simulink model "TV_Controller"  (R2019b)
settings: Solver=VariableStepAuto  StartTime=0.0  StopTime=10.0  RelTol=1e-3
values from neighbouring files (symbols this model uses):
  Kd_wheelSlip = 0    [runTorqueVectoringScript.m]
  Kd_yawController = 0    [runTorqueVectoringScript.m]
  Ki_wheelSlip = 0.1    [runTorqueVectoringScript.m]
  Ki_yawController = 0.1    [runTorqueVectoringScript.m]
  Kp_wheelSlip = 10    [runTorqueVectoringScript.m]
  Kp_yawController = 10    [runTorqueVectoringScript.m]
  lambda = 0.5    [runTorqueVectoringScript.m]
  Rd = 0.2    [runTorqueVectoringScript.m]
  ref_slip = 0.11    [runTorqueVectoringScript.m]
  tr = 1.1    [runTorqueVectoringScript.m]
libraries: simulink x5
settings Model: Creator=mha483  LastModifiedBy=mha483

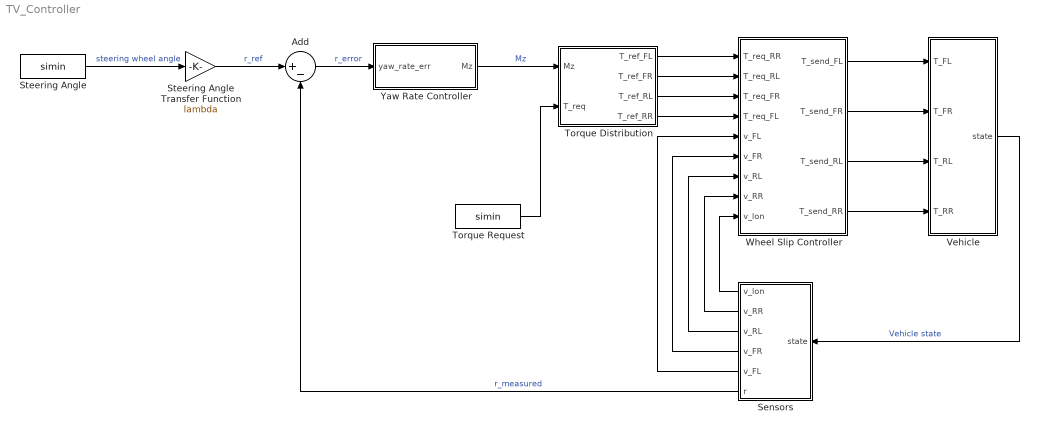
== system TV_Controller ==
  Add : Sum  Inputs=|+-
  Sensors : MATLAB Function  TreatAsAtomicUnit=on
  Steering Angle : FromWorkspace  VariableName=simin  SampleTime=0  Interpolate=off
  Steering Angle Transfer Function : Gain  Gain=lambda
  Torque Distribution : Subsystem
  Torque Request : FromWorkspace  VariableName=simin  SampleTime=0
  Vehicle : MATLAB Function  TreatAsAtomicUnit=on
  Wheel Slip Controller : Subsystem
  "Yaw Rate Controller " : Subsystem
  wires:
  "Yaw Rate Controller "/1(Mz) -> Torque Distribution/1(Mz)  "Mz"
  Torque Distribution/1(T_ref_FL) -> Wheel Slip Controller/1(T_req_RR)
  Torque Distribution/2(T_ref_FR) -> Wheel Slip Controller/2(T_req_RL)
  Torque Distribution/3(T_ref_RL) -> Wheel Slip Controller/3(T_req_FR)
  Torque Distribution/4(T_ref_RR) -> Wheel Slip Controller/4(T_req_FL)
  Add/1 -> "Yaw Rate Controller "/1(yaw_rate_err)  "r_error"
  Wheel Slip Controller/1(T_send_FL) -> Vehicle/1(T_FL)
  Wheel Slip Controller/2(T_send_FR) -> Vehicle/2(T_FR)
  Wheel Slip Controller/3(T_send_RL) -> Vehicle/3(T_RL)
  Wheel Slip Controller/4(T_send_RR) -> Vehicle/4(T_RR)
  Sensors/1(v_lon) -> Wheel Slip Controller/9(v_lon)
  Sensors/2(v_RR) -> Wheel Slip Controller/8(v_RR)
  Sensors/3(v_RL) -> Wheel Slip Controller/7(v_RL)
  Sensors/4(v_FR) -> Wheel Slip Controller/6(v_FR)
  Sensors/5(v_FL) -> Wheel Slip Controller/5(v_FL)
  Sensors/6(r) -> Add/2  "r_measured"
  Vehicle/1(state) -> Sensors/1(state)  "Vehicle state"
  Torque Request/1 -> Torque Distribution/2(T_req)
  Steering Angle Transfer Function/1 -> Add/1  "r_ref"
  Steering Angle/1 -> Steering Angle Transfer Function/1  "steering wheel angle"

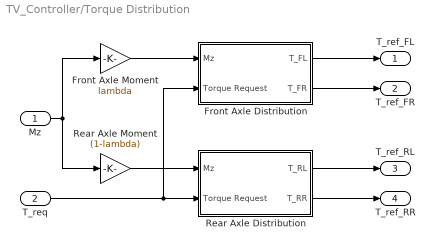
== system TV_Controller/Torque Distribution ==
  Mz : Inport
  T_req : Inport  Port=2
  Front Axle Moment : Gain  Gain=lambda
  Front Axle Distribution : Subsystem
  Rear Axle Moment : Gain  Gain=(1-lambda)
  Rear Axle Distribution : Subsystem
  T_ref_FL : Outport
  T_ref_FR : Outport  Port=2
  T_ref_RL : Outport  Port=3
  T_ref_RR : Outport  Port=4
  wires:
  Mz/1 -> Rear Axle Moment/1, Front Axle Moment/1
  Front Axle Moment/1 -> Front Axle Distribution/1(Mz)
  T_req/1 -> Rear Axle Distribution/2(Torque Request), Front Axle Distribution/2(Torque Request)
  Front Axle Distribution/2(T_FR) -> T_ref_FR/1
  Front Axle Distribution/1(T_FL) -> T_ref_FL/1
  Rear Axle Moment/1 -> Rear Axle Distribution/1(Mz)
  Rear Axle Distribution/1(T_RL) -> T_ref_RL/1
  Rear Axle Distribution/2(T_RR) -> T_ref_RR/1

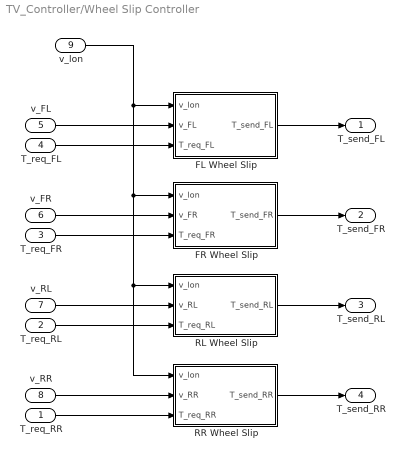
== system TV_Controller/Wheel Slip Controller ==
  T_req_RR : Inport
  T_req_RL : Inport  Port=2
  T_req_FR : Inport  Port=3
  T_req_FL : Inport  Port=4
  v_FL : Inport  Port=5
  v_FR : Inport  Port=6
  v_RL : Inport  Port=7
  v_RR : Inport  Port=8
  v_lon : Inport  Port=9
  FL Wheel Slip : Subsystem
  FR Wheel Slip : Subsystem
  RL Wheel Slip : Subsystem
  RR Wheel Slip : Subsystem
  T_send_FL : Outport
  T_send_FR : Outport  Port=2
  T_send_RL : Outport  Port=3
  T_send_RR : Outport  Port=4
  wires:
  v_lon/1 -> RR Wheel Slip/1(v_lon), RL Wheel Slip/1(v_lon), FR Wheel Slip/1(v_lon), FL Wheel Slip/1(v_lon)
  v_FL/1 -> FL Wheel Slip/2(v_FL)
  T_req_FL/1 -> FL Wheel Slip/3(T_req_FL)
  v_FR/1 -> FR Wheel Slip/2(v_FR)
  T_req_FR/1 -> FR Wheel Slip/3(T_req_FR)
  v_RL/1 -> RL Wheel Slip/2(v_RL)
  T_req_RL/1 -> RL Wheel Slip/3(T_req_RL)
  v_RR/1 -> RR Wheel Slip/2(v_RR)
  T_req_RR/1 -> RR Wheel Slip/3(T_req_RR)
  FL Wheel Slip/1(T_send_FL) -> T_send_FL/1
  FR Wheel Slip/1(T_send_FR) -> T_send_FR/1
  RL Wheel Slip/1(T_send_RL) -> T_send_RL/1
  RR Wheel Slip/1(T_send_RR) -> T_send_RR/1

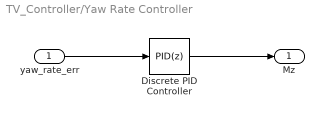
== system TV_Controller/Yaw Rate Controller  ==
  yaw_rate_err : Inport
  Discrete PID Controller : simulink/Continuous/PID Controller  Controller=PID  Form=Parallel  TimeDomain=Discrete-time  SampleTime=-1  IntegratorMethod=Forward Euler  FilterMethod=Forward Euler  ControllerParametersSource=internal  P=Kp_yawController  I=Ki_yawController  D=Kd_yawController  UseFilter=on  N=100  TunerSelectOption=Transfer Function Based (PID Tuner App)  InitialConditionSource=internal  InitialConditionForIntegrator=0  InitialConditionForFilter=0  DifferentiatorICPrevScaledInput=0  ExternalReset=none  TrackingMode=off  Kt=1  LimitOutput=off  UpperSaturationLimit=inf  LowerSaturationLimit=-inf  LinearizeAsGain=off  AntiWindupMode=none  Kb=1  POutMin=[]  POutMax=[]  IOutMin=[]  IOutMax=[]  DOutMin=[]  DOutMax=[]  NOutMin=[]  NOutMax=[]  SumOutMin=[]  SumOutMax=[]  SaturationOutMin=[]  SaturationOutMax=[]  PParamMin=[]  PParamMax=[]  IParamMin=[]  IParamMax=[]  DParamMin=[]  DParamMax=[]  NParamMin=[]  NParamMax=[]  KbParamMin=[]  KbParamMax=[]  KtParamMin=[]  KtParamMax=[]  KbOutMin=[]  KbOutMax=[]  KtOutMin=[]  KtOutMax=[]  IntegratorOutMin=[]  IntegratorOutMax=[]  FilterOutMin=[]  FilterOutMax=[]  SumI1OutMin=[]  SumI1OutMax=[]  SumI2OutMin=[]  SumI2OutMax=[]  SumI3OutMin=[]  SumI3OutMax=[]  SumI4OutMin=[]  SumI4OutMax=[]  SumDOutMin=[]  SumDOutMax=[]  DifferentiatorOutMin=[]  DifferentiatorOutMax=[]  FilterDiffOutCoefMin=[]  FilterDiffOutCoefMax=[]  ReciprocalOutMin=[]  ReciprocalOutMax=[]  SumDenOutMin=[]  SumDenOutMax=[]  SumNumOutMin=[]  SumNumOutMax=[]  DivideOutMin=[]  DivideOutMax=[]  IntegratorContinuousStateAttributes=''  IntegratorStateMustResolveToSignalObject=off  IntegratorRTWStateStorageClass=Auto  FilterContinuousStateAttributes=''  FilterStateMustResolveToSignalObject=off  FilterRTWStateStorageClass=Auto  ParallelPVariant=InternalParameters  IdealPVariant=Disabled  IVariant=InternalParameters  DVariant=InternalParameters  IntegratorVariant=Discrete  SatVariant=Disabled  AWVariant=Passthrough  PCopyVariant=Disabled  TRVariant=Disabled  FdbkBlocksVariant=Forward  IdealPFdbkVariant=Disabled  SatFdbkVariant=Disabled  DerivativeFilterVariant=ForwardEulerFilter  NVariant=InternalParameters  NCopyVariant=Disabled  FilterICVariant=InternalICsFilter  IntegratorICVariant=InternalICs  ExternalResetVariant=Disabled  TRSumVariant=Passthrough  SumFdbkVariant=Disabled  SumVariant=Sum_PID
  Mz : Outport
  wires:
  yaw_rate_err/1 -> Discrete PID Controller/1
  Discrete PID Controller/1 -> Mz/1

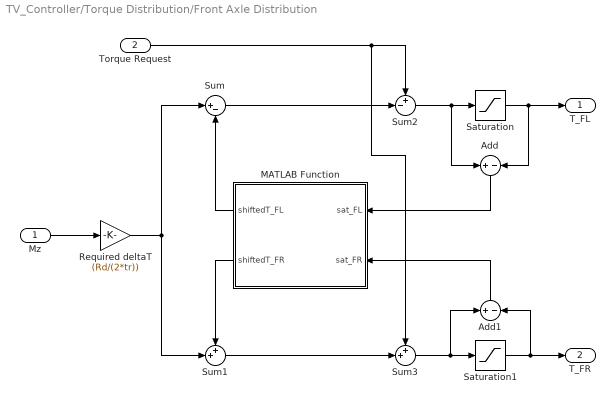
== system TV_Controller/Torque Distribution/Front Axle Distribution ==
  Mz : Inport
  Torque Request : Inport  Port=2
  Add : Sum  Inputs=+|-
  Add1 : Sum  Inputs=+|-
  MATLAB Function : MATLAB Function  TreatAsAtomicUnit=on
  Required deltaT : Gain  Gain=(Rd/(2*tr))
  Saturation : Saturate  UpperLimit=1000  LowerLimit=-1000
  Saturation1 : Saturate  UpperLimit=1000  LowerLimit=-1000
  Sum : Sum  Inputs=|+-
  Sum1 : Sum  Inputs=++|
  Sum2 : Sum  Inputs=+-|
  Sum3 : Sum  Inputs=++|
  T_FL : Outport
  T_FR : Outport  Port=2
  wires:
  Torque Request/1 -> Sum2/1, Sum3/1
  Saturation1/1 -> T_FR/1, Add1/2
  Saturation/1 -> T_FL/1, Add/2
  Sum3/1 -> Saturation1/1, Add1/1
  Sum2/1 -> Saturation/1, Add/1
  Sum1/1 -> Sum3/2
  Sum/1 -> Sum2/2
  Required deltaT/1 -> Sum/1, Sum1/2
  Mz/1 -> Required deltaT/1
  Add/1 -> MATLAB Function/1(sat_FL)
  Add1/1 -> MATLAB Function/2(sat_FR)
  MATLAB Function/1(shiftedT_FL) -> Sum/2
  MATLAB Function/2(shiftedT_FR) -> Sum1/1

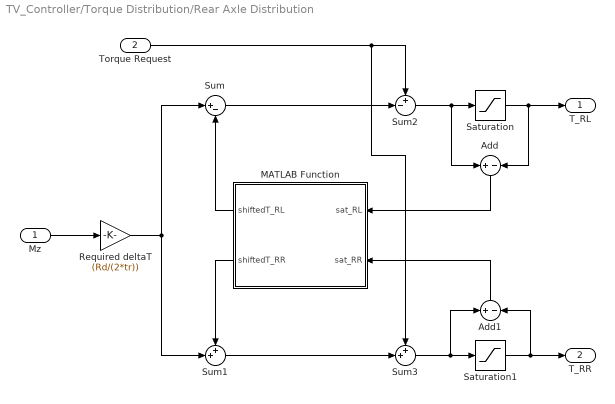
== system TV_Controller/Torque Distribution/Rear Axle Distribution ==
  Mz : Inport
  Torque Request : Inport  Port=2
  Add : Sum  Inputs=+|-
  Add1 : Sum  Inputs=+|-
  MATLAB Function : MATLAB Function  TreatAsAtomicUnit=on
  Required deltaT : Gain  Gain=(Rd/(2*tr))
  Saturation : Saturate  UpperLimit=1000  LowerLimit=-1000
  Saturation1 : Saturate  UpperLimit=1000  LowerLimit=-1000
  Sum : Sum  Inputs=|+-
  Sum1 : Sum  Inputs=++|
  Sum2 : Sum  Inputs=+-|
  Sum3 : Sum  Inputs=++|
  T_RL : Outport
  T_RR : Outport  Port=2
  wires:
  Required deltaT/1 -> Sum/1, Sum1/2
  Sum3/1 -> Saturation1/1, Add1/1
  Mz/1 -> Required deltaT/1
  Saturation1/1 -> T_RR/1, Add1/2
  Sum1/1 -> Sum3/2
  Sum/1 -> Sum2/2
  Saturation/1 -> T_RL/1, Add/2
  Torque Request/1 -> Sum2/1, Sum3/1
  Sum2/1 -> Saturation/1, Add/1
  Add1/1 -> MATLAB Function/2(sat_RR)
  Add/1 -> MATLAB Function/1(sat_RL)
  MATLAB Function/2(shiftedT_RR) -> Sum1/1
  MATLAB Function/1(shiftedT_RL) -> Sum/2

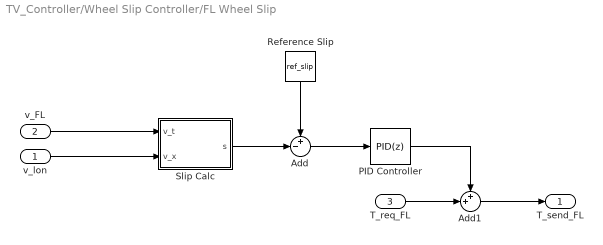
== system TV_Controller/Wheel Slip Controller/FL Wheel Slip ==
  v_lon : Inport
  v_FL : Inport  Port=2
  T_req_FL : Inport  Port=3
  Add : Sum  Inputs=+-|
  Add1 : Sum  Inputs=++|
  PID Controller : simulink/Continuous/PID Controller  Controller=PID  Form=Parallel  TimeDomain=Discrete-time  SampleTime=-1  IntegratorMethod=Forward Euler  FilterMethod=Forward Euler  ControllerParametersSource=internal  P=Kp_wheelSlip  I=Ki_wheelSlip  D=Kd_wheelSlip  UseFilter=on  N=100  TunerSelectOption=Transfer Function Based (PID Tuner App)  InitialConditionSource=internal  InitialConditionForIntegrator=0  InitialConditionForFilter=0  DifferentiatorICPrevScaledInput=0  ExternalReset=none  TrackingMode=off  Kt=1  LimitOutput=off  UpperSaturationLimit=inf  LowerSaturationLimit=-inf  LinearizeAsGain=on  AntiWindupMode=none  Kb=1  POutMin=[]  POutMax=[]  IOutMin=[]  IOutMax=[]  DOutMin=[]  DOutMax=[]  NOutMin=[]  NOutMax=[]  SumOutMin=[]  SumOutMax=[]  SaturationOutMin=[]  SaturationOutMax=[]  PParamMin=[]  PParamMax=[]  IParamMin=[]  IParamMax=[]  DParamMin=[]  DParamMax=[]  NParamMin=[]  NParamMax=[]  KbParamMin=[]  KbParamMax=[]  KtParamMin=[]  KtParamMax=[]  KbOutMin=[]  KbOutMax=[]  KtOutMin=[]  KtOutMax=[]  IntegratorOutMin=[]  IntegratorOutMax=[]  FilterOutMin=[]  FilterOutMax=[]  SumI1OutMin=[]  SumI1OutMax=[]  SumI2OutMin=[]  SumI2OutMax=[]  SumI3OutMin=[]  SumI3OutMax=[]  SumI4OutMin=[]  SumI4OutMax=[]  SumDOutMin=[]  SumDOutMax=[]  DifferentiatorOutMin=[]  DifferentiatorOutMax=[]  FilterDiffOutCoefMin=[]  FilterDiffOutCoefMax=[]  ReciprocalOutMin=[]  ReciprocalOutMax=[]  SumDenOutMin=[]  SumDenOutMax=[]  SumNumOutMin=[]  SumNumOutMax=[]  DivideOutMin=[]  DivideOutMax=[]  IntegratorContinuousStateAttributes=''  IntegratorStateMustResolveToSignalObject=off  IntegratorRTWStateStorageClass=Auto  FilterContinuousStateAttributes=''  FilterStateMustResolveToSignalObject=off  FilterRTWStateStorageClass=Auto  ParallelPVariant=InternalParameters  IdealPVariant=Disabled  IVariant=InternalParameters  DVariant=InternalParameters  IntegratorVariant=Discrete  SatVariant=Disabled  AWVariant=Passthrough  PCopyVariant=Disabled  TRVariant=Disabled  FdbkBlocksVariant=Forward  IdealPFdbkVariant=Disabled  SatFdbkVariant=Disabled  DerivativeFilterVariant=ForwardEulerFilter  NVariant=InternalParameters  NCopyVariant=Disabled  FilterICVariant=InternalICsFilter  IntegratorICVariant=InternalICs  ExternalResetVariant=Disabled  TRSumVariant=Passthrough  SumFdbkVariant=Disabled  SumVariant=Sum_PID
  "Reference Slip " : Constant  Value=ref_slip
  Slip Calc : MATLAB Function  TreatAsAtomicUnit=on
  T_send_FL : Outport
  wires:
  Add/1 -> PID Controller/1
  "Reference Slip "/1 -> Add/1
  Slip Calc/1(s) -> Add/2
  PID Controller/1 -> Add1/1
  T_req_FL/1 -> Add1/2
  Add1/1 -> T_send_FL/1
  v_lon/1 -> Slip Calc/2(v_x)
  v_FL/1 -> Slip Calc/1(v_t)

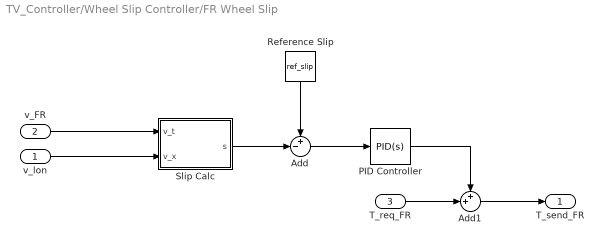
== system TV_Controller/Wheel Slip Controller/FR Wheel Slip ==
  v_lon : Inport
  v_FR : Inport  Port=2
  T_req_FR : Inport  Port=3
  Add : Sum  Inputs=+-|
  Add1 : Sum  Inputs=++|
  PID Controller : simulink/Continuous/PID Controller  Controller=PID  Form=Parallel  TimeDomain=Continuous-time  SampleTime=-1  IntegratorMethod=Forward Euler  FilterMethod=Forward Euler  ControllerParametersSource=internal  P=Kp_wheelSlip  I=Ki_wheelSlip  D=Kd_wheelSlip  UseFilter=on  N=100  TunerSelectOption=Transfer Function Based (PID Tuner App)  InitialConditionSource=internal  InitialConditionForIntegrator=0  InitialConditionForFilter=0  DifferentiatorICPrevScaledInput=0  ExternalReset=none  TrackingMode=off  Kt=1  LimitOutput=off  UpperSaturationLimit=inf  LowerSaturationLimit=-inf  LinearizeAsGain=on  AntiWindupMode=none  Kb=1  POutMin=[]  POutMax=[]  IOutMin=[]  IOutMax=[]  DOutMin=[]  DOutMax=[]  NOutMin=[]  NOutMax=[]  SumOutMin=[]  SumOutMax=[]  SaturationOutMin=[]  SaturationOutMax=[]  PParamMin=[]  PParamMax=[]  IParamMin=[]  IParamMax=[]  DParamMin=[]  DParamMax=[]  NParamMin=[]  NParamMax=[]  KbParamMin=[]  KbParamMax=[]  KtParamMin=[]  KtParamMax=[]  KbOutMin=[]  KbOutMax=[]  KtOutMin=[]  KtOutMax=[]  IntegratorOutMin=[]  IntegratorOutMax=[]  FilterOutMin=[]  FilterOutMax=[]  SumI1OutMin=[]  SumI1OutMax=[]  SumI2OutMin=[]  SumI2OutMax=[]  SumI3OutMin=[]  SumI3OutMax=[]  SumI4OutMin=[]  SumI4OutMax=[]  SumDOutMin=[]  SumDOutMax=[]  DifferentiatorOutMin=[]  DifferentiatorOutMax=[]  FilterDiffOutCoefMin=[]  FilterDiffOutCoefMax=[]  ReciprocalOutMin=[]  ReciprocalOutMax=[]  SumDenOutMin=[]  SumDenOutMax=[]  SumNumOutMin=[]  SumNumOutMax=[]  DivideOutMin=[]  DivideOutMax=[]  IntegratorContinuousStateAttributes=''  IntegratorStateMustResolveToSignalObject=off  IntegratorRTWStateStorageClass=Auto  FilterContinuousStateAttributes=''  FilterStateMustResolveToSignalObject=off  FilterRTWStateStorageClass=Auto  ParallelPVariant=InternalParameters  IdealPVariant=Disabled  IVariant=InternalParameters  DVariant=InternalParameters  IntegratorVariant=Continuous  SatVariant=Disabled  AWVariant=Passthrough  PCopyVariant=Disabled  TRVariant=Disabled  FdbkBlocksVariant=Forward  IdealPFdbkVariant=Disabled  SatFdbkVariant=Disabled  DerivativeFilterVariant=ContFilter  NVariant=InternalParameters  NCopyVariant=Disabled  FilterICVariant=InternalICsFilter  IntegratorICVariant=InternalICs  ExternalResetVariant=Disabled  TRSumVariant=Passthrough  SumFdbkVariant=Disabled  SumVariant=Sum_PID
  "Reference Slip " : Constant  Value=ref_slip
  Slip Calc : MATLAB Function  TreatAsAtomicUnit=on
  T_send_FR : Outport
  wires:
  Add/1 -> PID Controller/1
  "Reference Slip "/1 -> Add/1
  Slip Calc/1(s) -> Add/2
  PID Controller/1 -> Add1/1
  T_req_FR/1 -> Add1/2
  Add1/1 -> T_send_FR/1
  v_lon/1 -> Slip Calc/2(v_x)
  v_FR/1 -> Slip Calc/1(v_t)

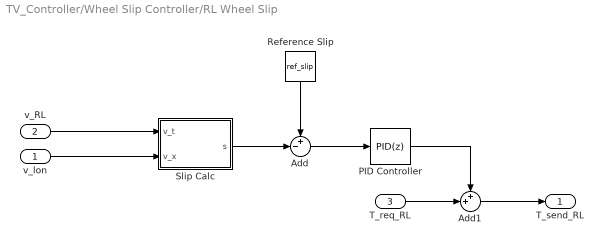
== system TV_Controller/Wheel Slip Controller/RL Wheel Slip ==
  v_lon : Inport
  v_RL : Inport  Port=2
  T_req_RL : Inport  Port=3
  Add : Sum  Inputs=+-|
  Add1 : Sum  Inputs=++|
  PID Controller : simulink/Continuous/PID Controller  Controller=PID  Form=Parallel  TimeDomain=Discrete-time  SampleTime=-1  IntegratorMethod=Forward Euler  FilterMethod=Forward Euler  ControllerParametersSource=internal  P=Kp_wheelSlip  I=Ki_wheelSlip  D=Kd_wheelSlip  UseFilter=on  N=100  TunerSelectOption=Transfer Function Based (PID Tuner App)  InitialConditionSource=internal  InitialConditionForIntegrator=0  InitialConditionForFilter=0  DifferentiatorICPrevScaledInput=0  ExternalReset=none  TrackingMode=off  Kt=1  LimitOutput=off  UpperSaturationLimit=inf  LowerSaturationLimit=-inf  LinearizeAsGain=on  AntiWindupMode=none  Kb=1  POutMin=[]  POutMax=[]  IOutMin=[]  IOutMax=[]  DOutMin=[]  DOutMax=[]  NOutMin=[]  NOutMax=[]  SumOutMin=[]  SumOutMax=[]  SaturationOutMin=[]  SaturationOutMax=[]  PParamMin=[]  PParamMax=[]  IParamMin=[]  IParamMax=[]  DParamMin=[]  DParamMax=[]  NParamMin=[]  NParamMax=[]  KbParamMin=[]  KbParamMax=[]  KtParamMin=[]  KtParamMax=[]  KbOutMin=[]  KbOutMax=[]  KtOutMin=[]  KtOutMax=[]  IntegratorOutMin=[]  IntegratorOutMax=[]  FilterOutMin=[]  FilterOutMax=[]  SumI1OutMin=[]  SumI1OutMax=[]  SumI2OutMin=[]  SumI2OutMax=[]  SumI3OutMin=[]  SumI3OutMax=[]  SumI4OutMin=[]  SumI4OutMax=[]  SumDOutMin=[]  SumDOutMax=[]  DifferentiatorOutMin=[]  DifferentiatorOutMax=[]  FilterDiffOutCoefMin=[]  FilterDiffOutCoefMax=[]  ReciprocalOutMin=[]  ReciprocalOutMax=[]  SumDenOutMin=[]  SumDenOutMax=[]  SumNumOutMin=[]  SumNumOutMax=[]  DivideOutMin=[]  DivideOutMax=[]  IntegratorContinuousStateAttributes=''  IntegratorStateMustResolveToSignalObject=off  IntegratorRTWStateStorageClass=Auto  FilterContinuousStateAttributes=''  FilterStateMustResolveToSignalObject=off  FilterRTWStateStorageClass=Auto  ParallelPVariant=InternalParameters  IdealPVariant=Disabled  IVariant=InternalParameters  DVariant=InternalParameters  IntegratorVariant=Discrete  SatVariant=Disabled  AWVariant=Passthrough  PCopyVariant=Disabled  TRVariant=Disabled  FdbkBlocksVariant=Forward  IdealPFdbkVariant=Disabled  SatFdbkVariant=Disabled  DerivativeFilterVariant=ForwardEulerFilter  NVariant=InternalParameters  NCopyVariant=Disabled  FilterICVariant=InternalICsFilter  IntegratorICVariant=InternalICs  ExternalResetVariant=Disabled  TRSumVariant=Passthrough  SumFdbkVariant=Disabled  SumVariant=Sum_PID
  "Reference Slip " : Constant  Value=ref_slip
  Slip Calc : MATLAB Function  TreatAsAtomicUnit=on
  T_send_RL : Outport
  wires:
  Add/1 -> PID Controller/1
  "Reference Slip "/1 -> Add/1
  Slip Calc/1(s) -> Add/2
  PID Controller/1 -> Add1/1
  T_req_RL/1 -> Add1/2
  Add1/1 -> T_send_RL/1
  v_lon/1 -> Slip Calc/2(v_x)
  v_RL/1 -> Slip Calc/1(v_t)

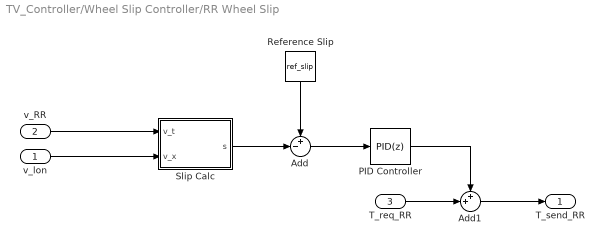
== system TV_Controller/Wheel Slip Controller/RR Wheel Slip ==
  v_lon : Inport
  v_RR : Inport  Port=2
  T_req_RR : Inport  Port=3
  Add : Sum  Inputs=+-|
  Add1 : Sum  Inputs=++|
  PID Controller : simulink/Continuous/PID Controller  Controller=PID  Form=Parallel  TimeDomain=Discrete-time  SampleTime=-1  IntegratorMethod=Forward Euler  FilterMethod=Forward Euler  ControllerParametersSource=internal  P=Kp_wheelSlip  I=Ki_wheelSlip  D=Kd_wheelSlip  UseFilter=on  N=100  TunerSelectOption=Transfer Function Based (PID Tuner App)  InitialConditionSource=internal  InitialConditionForIntegrator=0  InitialConditionForFilter=0  DifferentiatorICPrevScaledInput=0  ExternalReset=none  TrackingMode=off  Kt=1  LimitOutput=off  UpperSaturationLimit=inf  LowerSaturationLimit=-inf  LinearizeAsGain=on  AntiWindupMode=none  Kb=1  POutMin=[]  POutMax=[]  IOutMin=[]  IOutMax=[]  DOutMin=[]  DOutMax=[]  NOutMin=[]  NOutMax=[]  SumOutMin=[]  SumOutMax=[]  SaturationOutMin=[]  SaturationOutMax=[]  PParamMin=[]  PParamMax=[]  IParamMin=[]  IParamMax=[]  DParamMin=[]  DParamMax=[]  NParamMin=[]  NParamMax=[]  KbParamMin=[]  KbParamMax=[]  KtParamMin=[]  KtParamMax=[]  KbOutMin=[]  KbOutMax=[]  KtOutMin=[]  KtOutMax=[]  IntegratorOutMin=[]  IntegratorOutMax=[]  FilterOutMin=[]  FilterOutMax=[]  SumI1OutMin=[]  SumI1OutMax=[]  SumI2OutMin=[]  SumI2OutMax=[]  SumI3OutMin=[]  SumI3OutMax=[]  SumI4OutMin=[]  SumI4OutMax=[]  SumDOutMin=[]  SumDOutMax=[]  DifferentiatorOutMin=[]  DifferentiatorOutMax=[]  FilterDiffOutCoefMin=[]  FilterDiffOutCoefMax=[]  ReciprocalOutMin=[]  ReciprocalOutMax=[]  SumDenOutMin=[]  SumDenOutMax=[]  SumNumOutMin=[]  SumNumOutMax=[]  DivideOutMin=[]  DivideOutMax=[]  IntegratorContinuousStateAttributes=''  IntegratorStateMustResolveToSignalObject=off  IntegratorRTWStateStorageClass=Auto  FilterContinuousStateAttributes=''  FilterStateMustResolveToSignalObject=off  FilterRTWStateStorageClass=Auto  ParallelPVariant=InternalParameters  IdealPVariant=Disabled  IVariant=InternalParameters  DVariant=InternalParameters  IntegratorVariant=Discrete  SatVariant=Disabled  AWVariant=Passthrough  PCopyVariant=Disabled  TRVariant=Disabled  FdbkBlocksVariant=Forward  IdealPFdbkVariant=Disabled  SatFdbkVariant=Disabled  DerivativeFilterVariant=ForwardEulerFilter  NVariant=InternalParameters  NCopyVariant=Disabled  FilterICVariant=InternalICsFilter  IntegratorICVariant=InternalICs  ExternalResetVariant=Disabled  TRSumVariant=Passthrough  SumFdbkVariant=Disabled  SumVariant=Sum_PID
  "Reference Slip " : Constant  Value=ref_slip
  Slip Calc : MATLAB Function  TreatAsAtomicUnit=on
  T_send_RR : Outport
  wires:
  Add/1 -> PID Controller/1
  "Reference Slip "/1 -> Add/1
  Slip Calc/1(s) -> Add/2
  PID Controller/1 -> Add1/1
  T_req_RR/1 -> Add1/2
  Add1/1 -> T_send_RR/1
  v_lon/1 -> Slip Calc/2(v_x)
  v_RR/1 -> Slip Calc/1(v_t)

== matlab function TV_Controller/Wheel Slip Controller/RR Wheel Slip/Slip Calc ==
  data: v_t input; v_x input; s output
function s = fcn(v_t, v_x)

s = (v_t - v_x)/v_t;

== matlab function TV_Controller/Wheel Slip Controller/FL Wheel Slip/Slip Calc ==
  data: v_t input; v_x input; s output
function s = fcn(v_t, v_x)

s = (v_t - v_x)/v_t;

== matlab function TV_Controller/Wheel Slip Controller/RL Wheel Slip/Slip Calc ==
  data: v_t input; v_x input; s output
function s = fcn(v_t, v_x)

s = (v_t - v_x)/v_t;

== matlab function TV_Controller/Wheel Slip Controller/FR Wheel Slip/Slip Calc ==
  data: v_t input; v_x input; s output
function s = fcn(v_t, v_x)

s = (v_t - v_x)/v_t;

== matlab function TV_Controller/Torque Distribution/Front Axle Distribution/MATLAB Function ==
  data: sat_FL input; shiftedT_FL output; sat_FR input; shiftedT_FR output
function [shiftedT_FL,shiftedT_FR] = transferSaturatedTorqueFront(sat_FL,sat_FR)
% sends oversaturated parts of wheel torques to the opposite wheel,
% depending which wheel is more saturated.

% Function assumes the requested torques (from APPS) were within saturation
% limits before torque vectoring torques were applied

shiftedT_FL = 0;
shiftedT_FR = 0;

if sat_FL > sat_FR
    shiftedT_FR = sat_FL;
elseif sat_FL < sat_FR
    shiftedT_FL = sat_FR;
end

== matlab function TV_Controller/Torque Distribution/Rear Axle Distribution/MATLAB Function ==
  data: sat_RL input; shiftedT_RL output; sat_RR input; shiftedT_RR output
function [shiftedT_RL,shiftedT_RR] = transferSaturatedTorqueRear(sat_RL,sat_RR)
% sends oversaturated parts of wheel torques to the opposite wheel,
% depending which wheel is more saturated.

% Function assumes the requested torques (from APPS) were within saturation
% limits before torque vectoring torques were applied

shiftedT_RL = 0;
shiftedT_RR = 0;

if sat_FL > sat_RR
    shiftedT_RR = sat_RL;
elseif sat_FL < sat_RR
    shiftedT_RL = sat_RR;
end

== matlab function TV_Controller/Vehicle ==
  data: T_FL input; state output; T_FR input; T_RL input; T_RR input
function state = fcn(T_FL,T_FR,T_RL,T_RR)

y = u;

== matlab function TV_Controller/Sensors ==
  data: state input; v_lon output; v_RR output; v_RL output; v_FR output; v_FL output; r output
function [v_lon,v_RR,v_RL,v_FR,v_FL, r] = fcn(state)

y = u;
